simulink model "PID_Test"  (R2020b)
settings: Solver=VariableStepAuto  StartTime=0.0  StopTime=20  MaxStep=1e-4  RelTol=1e-3
libraries: pid_lib x1
settings Model: Creator=neilb  LastModifiedBy=neilb

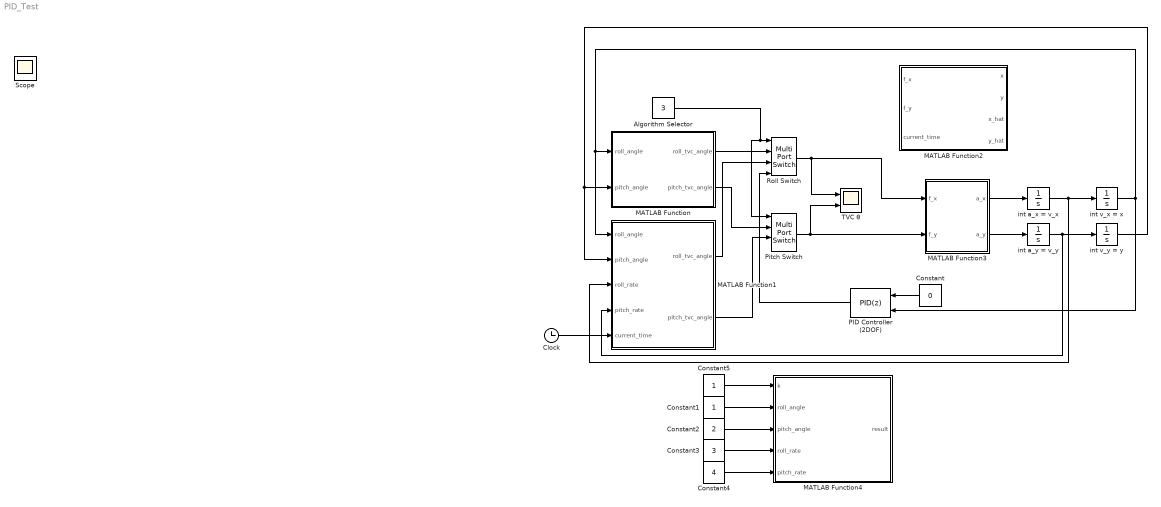
== system PID_Test ==
  Algorithm Selector : Constant  Value=3
  Clock : Clock
  Constant : Constant  Value=0
  Constant1 : Constant
  Constant2 : Constant  Value=2
  Constant3 : Constant  Value=3
  Constant4 : Constant  Value=4
  Constant5 : Constant
  MATLAB Function : MATLAB Function  TreatAsAtomicUnit=on
  MATLAB Function1 : MATLAB Function  TreatAsAtomicUnit=on
  MATLAB Function2 : MATLAB Function  TreatAsAtomicUnit=on
  MATLAB Function3 : MATLAB Function  TreatAsAtomicUnit=on
  MATLAB Function4 : MATLAB Function  TreatAsAtomicUnit=on
  PID Controller (2DOF) : pid_lib/PID Controller (2DOF)  Controller=PID  Form=Parallel  TimeDomain=Discrete-time  UseExternalTs=off  SampleTime=-1  IntegratorMethod=Forward Euler  FilterMethod=Forward Euler  ControllerParametersSource=internal  P=0.1  I=0.05  D=0.2  UseFilter=on  N=100  b=1  c=1  TunerSelectOption=Transfer Function Based (PID Tuner App)  InitialConditionSource=internal  InitialConditionForIntegrator=0  InitialConditionForFilter=0  DifferentiatorICPrevScaledInput=0  ExternalReset=none  TrackingMode=off  Kt=1  LimitOutput=off  SatLimitsSource=internal  UpperSaturationLimit=inf  LowerSaturationLimit=-inf  LinearizeAsGain=on  AntiWindupMode=none  Kb=1  POutMin=[]  POutMax=[]  IOutMin=[]  IOutMax=[]  DOutMin=[]  DOutMax=[]  NOutMin=[]  NOutMax=[]  bOutMin=[]  bOutMax=[]  cOutMin=[]  cOutMax=[]  SumOutMin=[]  SumOutMax=[]  SaturationOutMin=[]  SaturationOutMax=[]  PParamMin=[]  PParamMax=[]  IParamMin=[]  IParamMax=[]  DParamMin=[]  DParamMax=[]  NParamMin=[]  NParamMax=[]  bParamMin=[]  bParamMax=[]  cParamMin=[]  cParamMax=[]  KbParamMin=[]  KbParamMax=[]  KtParamMin=[]  KtParamMax=[]  KbOutMin=[]  KbOutMax=[]  KtOutMin=[]  KtOutMax=[]  IntegratorOutMin=[]  IntegratorOutMax=[]  FilterOutMin=[]  FilterOutMax=[]  SumI1OutMin=[]  SumI1OutMax=[]  SumI2OutMin=[]  SumI2OutMax=[]  SumI3OutMin=[]  SumI3OutMax=[]  SumI4OutMin=[]  SumI4OutMax=[]  SumDOutMin=[]  SumDOutMax=[]  Sum1OutMin=[]  Sum1OutMax=[]  Sum2OutMin=[]  Sum2OutMax=[]  Sum3OutMin=[]  Sum3OutMax=[]  DifferentiatorOutMin=[]  DifferentiatorOutMax=[]  FilterDiffOutCoefMin=[]  FilterDiffOutCoefMax=[]  ReciprocalOutMin=[]  ReciprocalOutMax=[]  SumDenOutMin=[]  SumDenOutMax=[]  SumNumOutMin=[]  SumNumOutMax=[]  DivideOutMin=[]  DivideOutMax=[]  UdiffTsProdOutMin=[]  UdiffTsProdOutMax=[]  NTsProdOutMin=[]  NTsProdOutMax=[]  UintegralTsProdOutMin=[]  UintegralTsProdOutMax=[]  UngainTsProdOutMin=[]  UngainTsProdOutMax=[]  IntegratorContinuousStateAttributes=''  IntegratorStateMustResolveToSignalObject=off  IntegratorRTWStateStorageClass=Auto  FilterContinuousStateAttributes=''  FilterStateMustResolveToSignalObject=off  FilterRTWStateStorageClass=Auto  ParallelPVariant=InternalParameters  IdealPVariant=Disabled  IVariant=InternalParameters  DVariant=InternalParameters  bVariant=InternalParameters  cVariant=InternalParameters  IntegratorVariant=Discrete  SatVariant=Disabled  AWVariant=Passthrough  PCopyVariant=Disabled  TRVariant=Disabled  FdbkBlocksVariant=Forward  IdealPFdbkVariant=Disabled  SatFdbkVariant=Disabled  DerivativeFilterVariant=ForwardEulerFilter  NVariant=InternalParameters  NCopyVariant=Disabled  FilterICVariant=InternalICsFilter  IntegratorICVariant=InternalICs  ExternalResetVariant=Disabled  TRSumVariant=Passthrough  SumFdbkVariant=Disabled  SumVariant=Sum_PID  TsampFilterVariant=InternalTs  TsampNgainVariant=Passthrough  TsampIntegralVariant=Passthrough  ExternalSaturationOutDataTypeStr=Inherit: Same as second input
      settings: SourceProductBaseCode=SL
  Pitch Switch : MultiPortSwitch
  Roll Switch : MultiPortSwitch
  TVC θ : Scope  NumInputPorts=2
  int a_x = v_x : Integrator
  int a_y = v_y : Integrator
  int v_x = x : Integrator  InitialCondition=50
  int v_y = y : Integrator  InitialCondition=25
  Scope : Scope
  wires:
  MATLAB Function1/2(pitch_tvc_angle) -> Pitch Switch/3
  MATLAB Function1/1(roll_tvc_angle) -> Roll Switch/3
  Clock/1 -> MATLAB Function1/5(current_time)
  MATLAB Function/2(pitch_tvc_angle) -> Pitch Switch/2
  MATLAB Function/1(roll_tvc_angle) -> Roll Switch/2
  Algorithm Selector/1 -> Pitch Switch/1, Roll Switch/1
  Roll Switch/1 -> TVC θ/1, MATLAB Function3/1(f_x)
  Pitch Switch/1 -> MATLAB Function3/2(f_y), TVC θ/2
  MATLAB Function3/1(a_x) -> int a_x = v_x/1
  MATLAB Function3/2(a_y) -> int a_y = v_y/1
  int a_y = v_y/1 -> MATLAB Function1/4(pitch_rate), int v_y = y/1
  int a_x = v_x/1 -> MATLAB Function1/3(roll_rate), int v_x = x/1
  int v_x = x/1 -> PID Controller (2DOF)/2, MATLAB Function1/1(roll_angle), MATLAB Function/1(roll_angle)
  int v_y = y/1 -> MATLAB Function/2(pitch_angle), MATLAB Function1/2(pitch_angle)
  PID Controller (2DOF)/1 -> Roll Switch/4
  Constant/1 -> PID Controller (2DOF)/1
  Constant1/1 -> MATLAB Function4/2(roll_angle)
  Constant2/1 -> MATLAB Function4/3(pitch_angle)
  Constant3/1 -> MATLAB Function4/4(roll_rate)
  Constant4/1 -> MATLAB Function4/5(pitch_rate)
  Constant5/1 -> MATLAB Function4/1(k)

== matlab function PID_Test/MATLAB Function1 ==
  settings: updateMethod=DISCRETE
  data: roll_angle input; roll_tvc_angle output; pitch_angle input; roll_rate input; pitch_rate input; pitch_tvc_angle output; current_time input
function [roll_tvc_angle, pitch_tvc_angle] = pid_controller(roll_angle, pitch_angle, roll_rate, pitch_rate, current_time)
    %This function calculates an appropriate 2D tvc command using a 
    % PID-controller and the current deviation from vertical flight.
    p_gain = 0.1;
    i_gain = 0.05;
    d_gain = 0.2;
    
    roll_error = -roll_angle;
    pitch_error = -pitch_angle;
    
    % Persistent Variables are remembered between function calls (https://www.mathworks.com/help/matlab/ref/persistent.html)
    persistent last_time;
    if isempty(last_time)
        last_time = 0;
    end
    dt = current_time - last_time;
    persistent sum_roll_error;
    if isempty(sum_roll_error)
        sum_roll_error = 0;
    else
        sum_roll_error = sum_roll_error + dt * roll_error;
    end

    persistent sum_pitch_error;
    if isempty(sum_pitch_error)
        sum_pitch_error = 0;
    else
        sum_pitch_error = sum_pitch_error + dt * pitch_error;
    end
    last_time = current_time;
    
    % https://en.wikipedia.org/wiki/PID_controller#Mathematical_form
    roll_tvc_angle = p_gain * roll_error + i_gain * sum_roll_error + d_gain * roll_rate;
    pitch_tvc_angle = p_gain * pitch_error + i_gain * sum_pitch_error + d_gain * pitch_rate;
    % Uncomment the following line to use column vector output.
    %tvc_angle = [roll_tvc_angle; pitch_tvc_angle];
end

== matlab function PID_Test/MATLAB Function ==
  data: roll_angle input; roll_tvc_angle output; pitch_angle input; pitch_tvc_angle output
function [roll_tvc_angle, pitch_tvc_angle] = p_controller(roll_angle, pitch_angle)
    %This function calculates an appropriate 2D tvc command using a 
    % P-controller and the current deviation from vertical flight.
    p_gain_tvc_attitude_correction = 0.5;
    
    % The tvc angle should be opposite the current roll angle to apply a
    % corrective/normalizing torque.
    roll_tvc_angle = - p_gain_tvc_attitude_correction * roll_angle;
    pitch_tvc_angle = - p_gain_tvc_attitude_correction * pitch_angle;
    % Uncomment the following line to use column vector output.
    %tvc_angle = [roll_tvc_angle; pitch_tvc_angle];
end

== matlab function PID_Test/MATLAB Function2 ==
  settings: updateMethod=DISCRETE
  data: x output; f_x input; y output; f_y input; x_hat output; y_hat output; current_time input
function [x, y, x_hat, y_hat] = point_mass(f_x, f_y, current_time)
    % Persistent Variables are remembered between function calls (https://www.mathworks.com/help/matlab/ref/persistent.html)
    persistent last_time;
    if isempty(last_time)
        last_time = 0;
    end
    persistent v_x;
    if isempty(v_x)
        v_x = 0;
    end
    persistent v_y;
    if isempty(v_y)
        v_y = 0;
    end
    persistent x_pos;
    if isempty(x_pos)
        x_pos = 0;
    end
    persistent y_pos;
    if isempty(y_pos)
        y_pos = 0;
    end
    
    dt = current_time - last_time;
    m = 3; % kg
    a_x = f_x / m;
    a_y = f_y / m;
    v_x = v_x + a_x * dt;
    v_y = v_y + a_y * dt;
    x_pos = x_pos + v_x * dt;
    y_pos = y_pos + v_y * dt;

    last_time = current_time;
    x_hat = v_x;
    y_hat = v_y;
    x = x_pos;
    y = y_pos;

== matlab function PID_Test/MATLAB Function3 ==
  data: f_x input; a_x output; f_y input; a_y output
function [a_x, a_y] = f_to_a(f_x, f_y)
    m = 5; % kg
    a_x = f_x / m;
    a_y = f_y / m;

== matlab function PID_Test/MATLAB Function4 ==
  data: k input; result output; roll_angle input; pitch_angle input; roll_rate input; pitch_rate input
function result = k_by_mat(k, roll_angle, pitch_angle, roll_rate, pitch_rate)
    mult = [roll_angle; pitch_angle; roll_rate; pitch_rate];
    result = k * mult;
